simulink model "ScpAp_VechileLongiControl"  (R2025b)
settings: Solver=FixedStepDiscrete  StartTime=0.0  StopTime=10.0  FixedStep=0.01  RelTol=1e-3
undefined symbols (not defined in the file): DT, Ki, Kp, SafetyMode_L2p_IDT
settings Model: DataDictionary=EgasPOC.sldd  Creator=IAST283  LastModifiedBy=IAST283
settings DataIOCC: SaveFormat=StructureWithTime
settings OptimizationCC: DefaultParameterBehavior=Inlined  EnhancedBackFolding=on  PassReuseOutputArgsAs=Individual arguments  ZeroExternalMemoryAtStartup=off  ZeroInternalMemoryAtStartup=off  OptimizeBlockOrder=speed  DifferentSizesBufferReuse=on  OptimizationCustomize=off  EfficientTunableParamExpr=on
settings DebuggingCC: ParameterTunabilityLossMsg=error
settings SFSimCC: MATLABDynamicMemAlloc=off
settings RTWCC: SystemTargetFile=autosar.tlc  GenCodeOnly=on  TemplateMakefile=ert_default_tmf  DataTypeReplacement=CDataTypesFixedWidth  Description=AUTOSAR
settings CodeAppCC: ForceParamTrailComments=on  IgnoreCustomStorageClasses=off  OperatorAnnotations=on  SimulinkDataObjDesc=on  SFDataObjDesc=on  InsertBlockDesc=on
settings STFCustomTargetCC: SystemTargetFile=autosar.tlc  TargetLangStandard=C99 (ISO)  MultiwordLength=256.0  ParMdlRefBuildCompliant=on  CompOptLevelCompliant=on  ConcurrentExecutionCompliant=off  IncludeMdlTerminateFcn=off  CombineOutputUpdateFcns=on  SuppressErrorStatus=on  ERTCustomFileBanners=on  SupportNonFinite=off  SupportComplex=off  SupportContinuousTime=off  SupportNonInlinedSFcns=off  RemoveResetFunc=on  MATLABClassNameForMDSCustomization=Simulink.SoftwareTarget.ERTCustomization  AutosarCompliant=on  GRTInterface=off  UseToolchainInfoCompliant=on  LookupTableObjectStructAxisOrder=2,1,3,4,...  LUTObjectStructOrderEvenSpacing=Size,Table,Breakpoints  AutosarMatrixIOAsArray=off  AutosarSchemaVersion=R20-11  AutosarCompilerAbstraction=off  DisableAUTOSARRoutinesHostLibrary=off  AutosarMaxShortNameLength=128.0
settings ERTTargetCC: ERTCustomFileTemplate=example_file_process.tlc  BooleanTrueId=TRUE  BooleanFalseId=FALSE  TargetLangStandard=C99 (ISO)  ConcurrentExecutionCompliant=off  IncludeMdlTerminateFcn=off  SuppressErrorStatus=on  SupportNonFinite=off  SupportComplex=off  ModelStepFunctionPrototypeControlCompliant=off  CPPClassGenCompliant=off  AutosarCompliant=on  LookupTableObjectStructAxisOrder=2,1,3,4,...  LUTObjectStructOrderEvenSpacing=Size,Table,Breakpoints

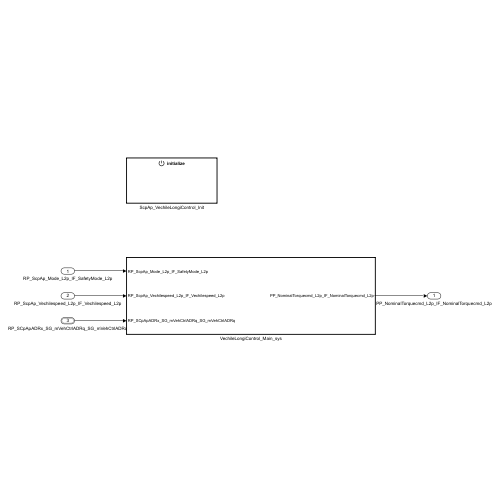
[thumbnail: Simulink's stored preview of the top-level diagram]
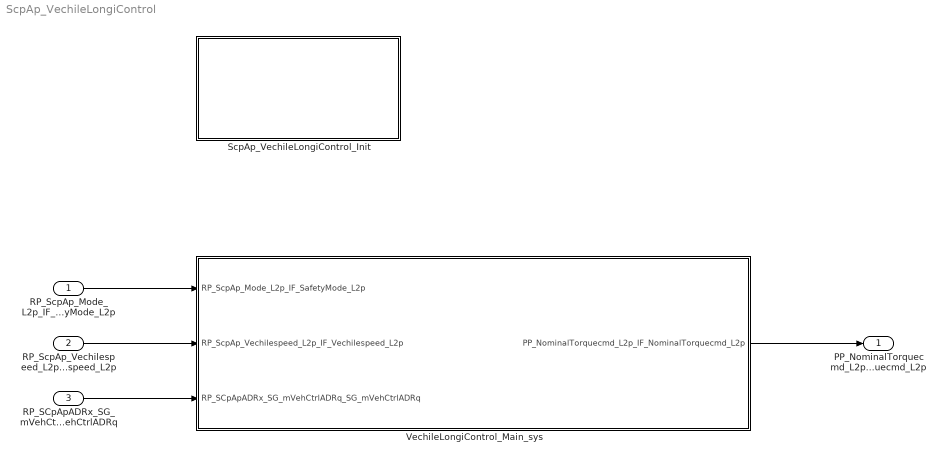
== system ScpAp_VechileLongiControl ==
  RP_ScpAp_Mode_L2p_IF_SafetyMode_L2p : Inport  OutDataTypeStr=Enum: SafetyMode_L2p_IDT  PortDimensions=1
  RP_ScpAp_Vechilespeed_L2p_IF_Vechilespeed_L2p : Inport  Port=2  OutDataTypeStr=uint16  PortDimensions=1
  RP_SCpApADRx_SG_mVehCtrlADRq_SG_mVehCtrlADRq : Inport  Port=3  OutDataTypeStr=Bus: SG_mVehCtrlADRq_IDT_E2E  PortDimensions=1  BusOutputAsStruct=on
  ScpAp_VechileLongiControl_Init : Subsystem
  VechileLongiControl_Main_sys : Subsystem  TreatAsAtomicUnit=on  SystemSampleTime=0.01
  PP_NominalTorquecmd_L2p_IF_NominalTorquecmd_L2p : Outport  OutDataTypeStr=int16  PortDimensions=1
  wires:
  RP_ScpAp_Mode_L2p_IF_SafetyMode_L2p/1 -> VechileLongiControl_Main_sys/1(RP_ScpAp_Mode_L2p_IF_SafetyMode_L2p)
  RP_ScpAp_Vechilespeed_L2p_IF_Vechilespeed_L2p/1 -> VechileLongiControl_Main_sys/2(RP_ScpAp_Vechilespeed_L2p_IF_Vechilespeed_L2p)
  RP_SCpApADRx_SG_mVehCtrlADRq_SG_mVehCtrlADRq/1 -> VechileLongiControl_Main_sys/3(RP_SCpApADRx_SG_mVehCtrlADRq_SG_mVehCtrlADRq)
  VechileLongiControl_Main_sys/1(PP_NominalTorquecmd_L2p_IF_NominalTorquecmd_L2p) -> PP_NominalTorquecmd_L2p_IF_NominalTorquecmd_L2p/1

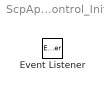
== system ScpAp_VechileLongiControl/ScpAp_VechileLongiControl_Init ==
  Event Listener : EventListener  EventName=reset

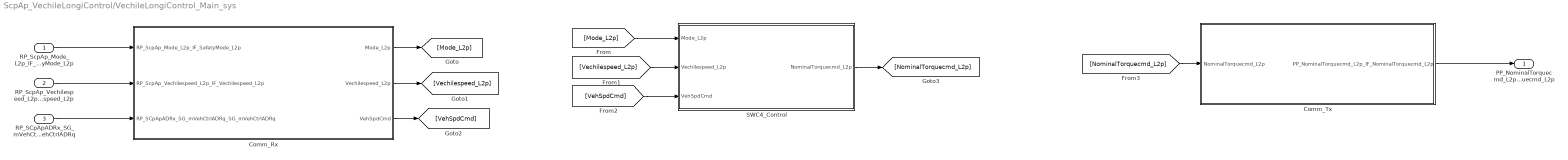
== system ScpAp_VechileLongiControl/VechileLongiControl_Main_sys ==
  RP_ScpAp_Mode_L2p_IF_SafetyMode_L2p : Inport  OutDataTypeStr=Enum: SafetyMode_L2p_IDT
  RP_ScpAp_Vechilespeed_L2p_IF_Vechilespeed_L2p : Inport  Port=2
  RP_SCpApADRx_SG_mVehCtrlADRq_SG_mVehCtrlADRq : Inport  Port=3
  Comm_Rx : Subsystem
  Comm_Tx : Subsystem
  SWC4_Control : Subsystem  TreatAsAtomicUnit=on
  PP_NominalTorquecmd_L2p_IF_NominalTorquecmd_L2p : Outport
  wires:
  RP_ScpAp_Mode_L2p_IF_SafetyMode_L2p/1 -> Comm_Rx/1(RP_ScpAp_Mode_L2p_IF_SafetyMode_L2p)
  RP_ScpAp_Vechilespeed_L2p_IF_Vechilespeed_L2p/1 -> Comm_Rx/2(RP_ScpAp_Vechilespeed_L2p_IF_Vechilespeed_L2p)
  RP_SCpApADRx_SG_mVehCtrlADRq_SG_mVehCtrlADRq/1 -> Comm_Rx/3(RP_SCpApADRx_SG_mVehCtrlADRq_SG_mVehCtrlADRq)
  Comm_Rx/1(Mode_L2p) -> [Mode_L2p]
  Comm_Rx/2(Vechilespeed_L2p) -> [Vechilespeed_L2p]
  Comm_Rx/3(VehSpdCmd) -> [VehSpdCmd]
  [Mode_L2p] -> SWC4_Control/1(Mode_L2p)
  [Vechilespeed_L2p] -> SWC4_Control/2(Vechilespeed_L2p)
  [VehSpdCmd] -> SWC4_Control/3(VehSpdCmd)
  SWC4_Control/1(NominalTorquecmd_L2p) -> [NominalTorquecmd_L2p]
  Comm_Tx/1(PP_NominalTorquecmd_L2p_IF_NominalTorquecmd_L2p) -> PP_NominalTorquecmd_L2p_IF_NominalTorquecmd_L2p/1
  [NominalTorquecmd_L2p] -> Comm_Tx/1(NominalTorquecmd_L2p)

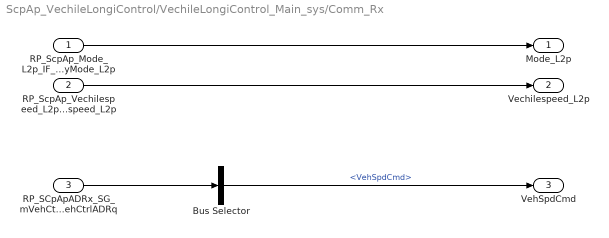
== system ScpAp_VechileLongiControl/VechileLongiControl_Main_sys/Comm_Rx ==
  RP_ScpAp_Mode_L2p_IF_SafetyMode_L2p : Inport  OutDataTypeStr=Enum: SafetyMode_L2p_IDT
  RP_ScpAp_Vechilespeed_L2p_IF_Vechilespeed_L2p : Inport  Port=2
  RP_SCpApADRx_SG_mVehCtrlADRq_SG_mVehCtrlADRq : Inport  Port=3
  Bus Selector : BusSelector  OutputSignals=VehSpdCmd
  Mode_L2p : Outport  OutDataTypeStr=Enum: SafetyMode_L2p_IDT
  Vechilespeed_L2p : Outport  Port=2
  VehSpdCmd : Outport  Port=3
  wires:
  Bus Selector/1 -> VehSpdCmd/1  "<VehSpdCmd>"
  RP_ScpAp_Mode_L2p_IF_SafetyMode_L2p/1 -> Mode_L2p/1
  RP_ScpAp_Vechilespeed_L2p_IF_Vechilespeed_L2p/1 -> Vechilespeed_L2p/1
  RP_SCpApADRx_SG_mVehCtrlADRq_SG_mVehCtrlADRq/1 -> Bus Selector/1

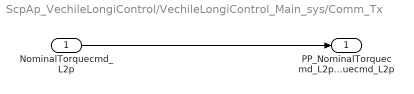
== system ScpAp_VechileLongiControl/VechileLongiControl_Main_sys/Comm_Tx ==
  NominalTorquecmd_L2p : Inport
  PP_NominalTorquecmd_L2p_IF_NominalTorquecmd_L2p : Outport
  wires:
  NominalTorquecmd_L2p/1 -> PP_NominalTorquecmd_L2p_IF_NominalTorquecmd_L2p/1

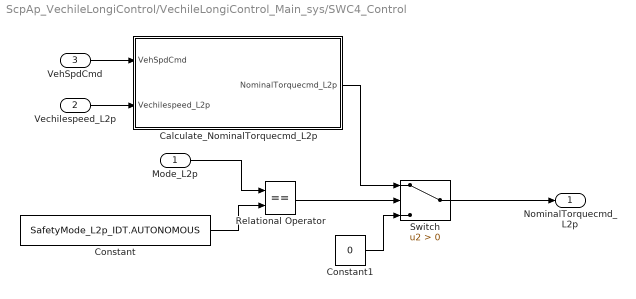
== system ScpAp_VechileLongiControl/VechileLongiControl_Main_sys/SWC4_Control ==
  Mode_L2p : Inport  OutDataTypeStr=Enum: SafetyMode_L2p_IDT
  Vechilespeed_L2p : Inport  Port=2
  VehSpdCmd : Inport  Port=3
  Calculate_NominalTorquecmd_L2p : Subsystem
  Constant : Constant  Value=SafetyMode_L2p_IDT.AUTONOMOUS  OutDataTypeStr=Enum: SafetyMode_L2p_IDT
  Constant1 : Constant  Value=0  OutDataTypeStr=boolean
  Relational Operator : RelationalOperator  Operator===  OutDataTypeStr=boolean  RndMeth=Simplest  InputSameDT=off
  Switch : Switch  Criteria=u2 > Threshold  SaturateOnIntegerOverflow=off  InputSameDT=off
  NominalTorquecmd_L2p : Outport
  wires:
  Relational Operator/1 -> Switch/2
  Mode_L2p/1 -> Relational Operator/1
  Switch/1 -> NominalTorquecmd_L2p/1
  Constant1/1 -> Switch/3
  Vechilespeed_L2p/1 -> Calculate_NominalTorquecmd_L2p/2(Vechilespeed_L2p)
  VehSpdCmd/1 -> Calculate_NominalTorquecmd_L2p/1(VehSpdCmd)
  Calculate_NominalTorquecmd_L2p/1(NominalTorquecmd_L2p) -> Switch/1
  Constant/1 -> Relational Operator/2

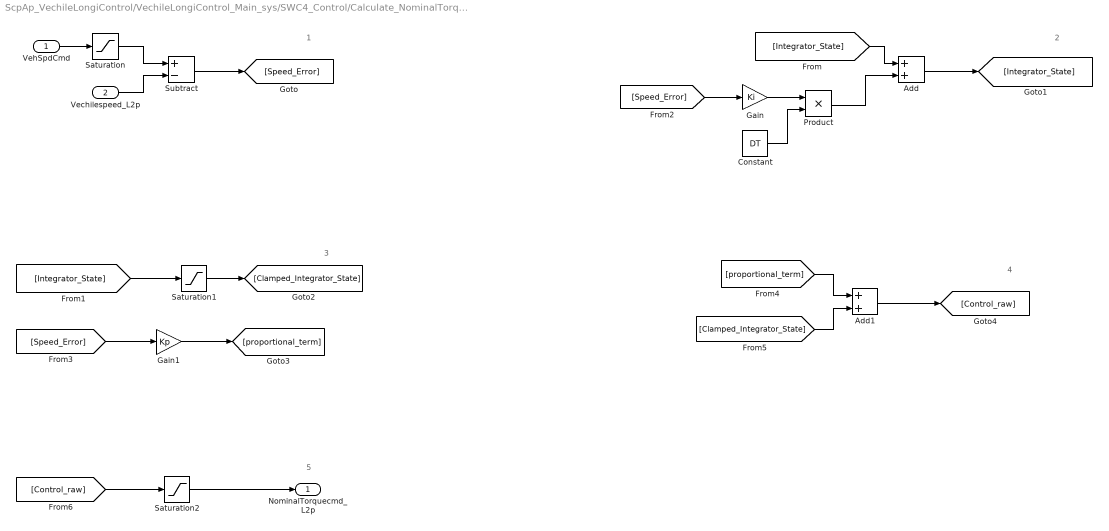
== system ScpAp_VechileLongiControl/VechileLongiControl_Main_sys/SWC4_Control/Calculate_NominalTorquecmd_L2p ==
  note: 5
  note: 4
  note: 3
  note: 2
  note: 1
  VehSpdCmd : Inport
  Vechilespeed_L2p : Inport  Port=2
  Add : Sum
  Add1 : Sum  OutDataTypeStr=int16
  Constant : Constant  Value=DT
  Gain : Gain  Gain=Ki
  Gain1 : Gain  Gain=Kp
  Product : Product
  Saturation : Saturate  UpperLimit=32  LowerLimit=0
  Saturation1 : Saturate  UpperLimit=30  LowerLimit=-30
  Saturation2 : Saturate  UpperLimit=120  LowerLimit=-70
  Subtract : Sum  Inputs=+-
  NominalTorquecmd_L2p : Outport
  wires:
  VehSpdCmd/1 -> Saturation/1
  Saturation/1 -> Subtract/1
  Vechilespeed_L2p/1 -> Subtract/2
  Subtract/1 -> [Speed_Error]
  Add/1 -> [Integrator_State]
  [Integrator_State] -> Add/1
  [Speed_Error] -> Gain/1
  Gain/1 -> Product/1
  Constant/1 -> Product/2
  Product/1 -> Add/2
  [Integrator_State] -> Saturation1/1
  Saturation1/1 -> [Clamped_Integrator_State]
  [Speed_Error] -> Gain1/1
  Gain1/1 -> [proportional_term]
  Add1/1 -> [Control_raw]
  [proportional_term] -> Add1/1
  [Clamped_Integrator_State] -> Add1/2
  [Control_raw] -> Saturation2/1
  Saturation2/1 -> NominalTorquecmd_L2p/1
